simulink model "DCMotorVal"  (R2025a)
settings: Solver=ode23s  StartTime=0.0  StopTime=10  RelTol=1e-3
undefined symbols (not defined in the file): rev_comms_sink
settings Model: Creator=jmp8430  LastModifiedBy=jmp8430

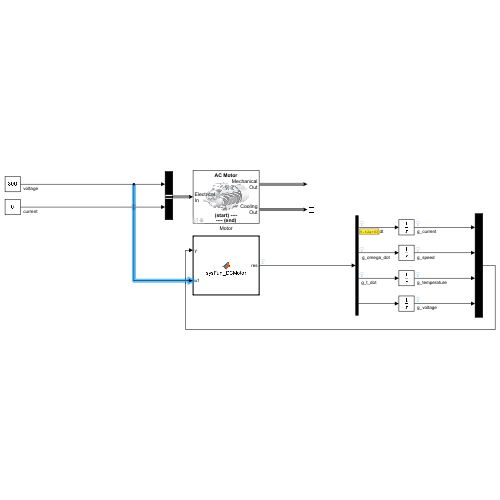
[thumbnail: Simulink's stored preview of the top-level diagram]
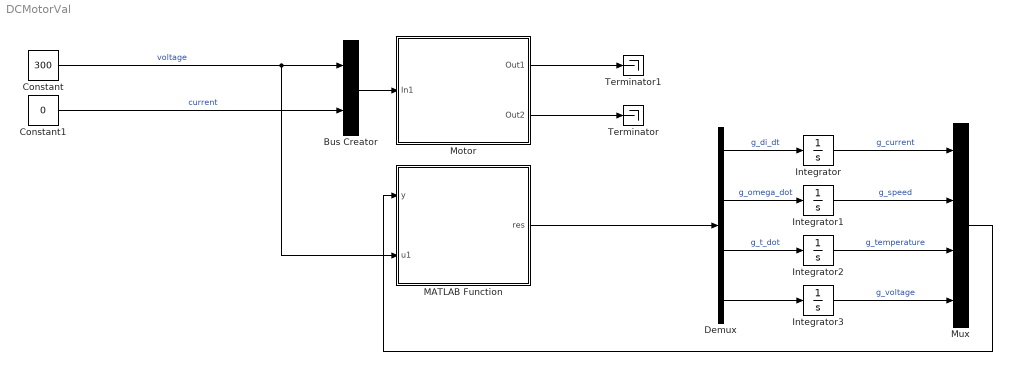
== system DCMotorVal ==
  Bus Creator : BusCreator  Inputs=2
  Constant : Constant  Value=300
  Constant1 : Constant  Value=0
  Demux : Demux
  Integrator : Integrator  InitialCondition=1
  Integrator1 : Integrator  InitialCondition=1
  Integrator2 : Integrator  InitialCondition=25
  Integrator3 : Integrator  InitialCondition=25
  MATLAB Function : MATLAB Function  TreatAsAtomicUnit=on
  Motor : Subsystem  AncestorBlock=DAEMOT_Lib/Electrical/Motor  mask{m_type=AC, R=0.013461960749493, Kv=0.009688163543703, c=0.000234355495215172, b=1.89435163576232e-05, L=1.252192537082724e-05, J=1.09*10^-4, I_initial=1, w_initial=1, Cp=60, T_initial=25}
      mask prompts: m_type "Motor Type"; R "Armature Resistance [Ohm]"; Kv "Motor Constant [Nm/A] or [V-s/rad]"; c "Static Friction Coefficient [Nm]"; b "Viscous Friction Coefficient [N*m*s/rad]"; L "Armature Inductance [H]"; J "Shaft Inertia [kg*m^2]"; I_initial "Initial Total Current [A]"; w_initial "Initial Speed [rad/s]"; Cp "Motor Heat Capacity [J/K]"; T_initial "Initial Temperature [C]"
      settings: LibrarySourceBlock=DAEMOT_Lib_Copy/Dyn Electrical Comp/Motor
      settings: CopyFcn=|
      | h      = get_param(gcb,'handle');   % Get block handle
      | blk    = gcb;
      | 
      | set_param(blk, 'LinkStatus', 'inactive')
      | clear h
      | clear blk
      mask TypeOptions m_type: DC | AC
      mask DialogControl ParameterTabVar0 Prompt: Motor Parameters
      mask DialogControl ParameterTabVar01 Prompt: Cooling
      mask DialogControl ParameterTabVar012 Prompt: System
      mask Display:
      | image(imread('motor.bmp'));
      | T = get_param(gcb,'m_type');
      | if strcmp(T,'DC')
      |     text(0.5,0.95,['{\bf DC Motor}'],'TexMode','on','horizontalAlignment', 'center')
      | else
      |     text(0.5,0.95,['{\bf AC Motor}'],'TexMode','on','horizontalAlignment', 'center')
      | end
      | text(0.5,0.075,['{\bf ---- (end)}'],'TexMode','on','horizontalAlignment', 'center')
      | text(0.5,0.175,['{\bf (start) ----}'],'TexMode','on','horizontalAlignment', 'center')
      | 
      | port_label('input',1,sprintf('Electrical \nIn'))
      | port_label('output',1,sprintf('Mechanical \nOut'))
      | port_label('output',2,sprintf('Cooling \nOut'))
  Mux : Mux
  Terminator : Terminator
  Terminator1 : Terminator
  wires:
  MATLAB Function/1(res) -> Demux/1
  Motor/2(Out2) -> Terminator/1
  Motor/1(Out1) -> Terminator1/1
  Constant/1 -> MATLAB Function/2(u1), Bus Creator/1  "voltage"
  Bus Creator/1 -> Motor/1(In1)
  Constant1/1 -> Bus Creator/2  "current"
  Demux/1 -> Integrator/1  "g_di_dt"
  Demux/2 -> Integrator1/1  "g_omega_dot"
  Demux/3 -> Integrator2/1  "g_t_dot"
  Demux/4 -> Integrator3/1
  Integrator/1 -> Mux/1  "g_current"
  Integrator1/1 -> Mux/2  "g_speed"
  Integrator2/1 -> Mux/3  "g_temperature"
  Mux/1 -> MATLAB Function/1(y)
  Integrator3/1 -> Mux/4  "g_voltage"

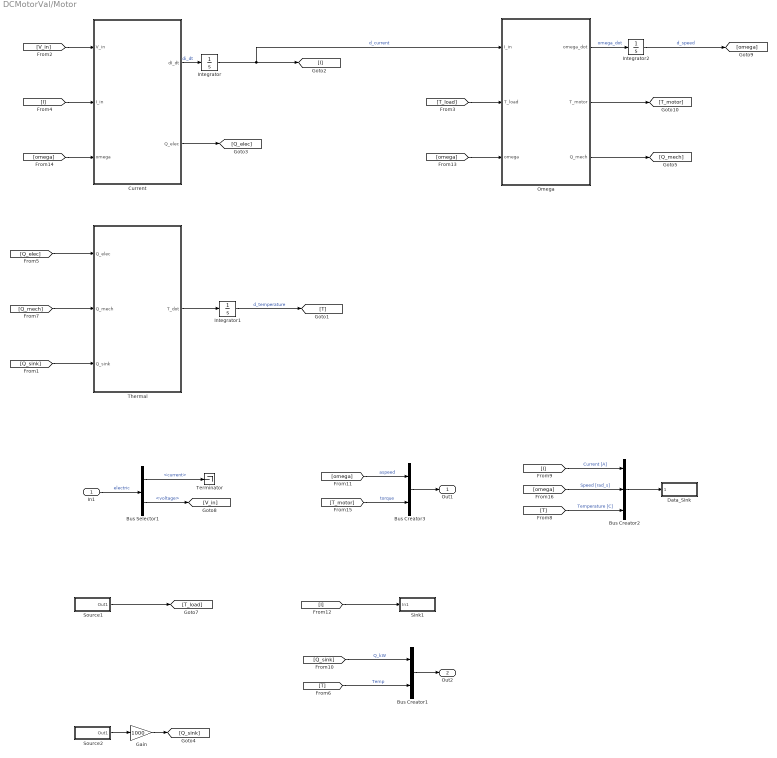
== system DCMotorVal/Motor ==
  In1 : Inport
  Bus Creator1 : BusCreator  Inputs=2
  Bus Creator2 : BusCreator  Inputs=3
  Bus Creator3 : BusCreator  Inputs=2
  Bus Selector1 : BusSelector  OutputSignals=current,voltage
  Current : MATLAB Function  TreatAsAtomicUnit=on
  Data_Sink : Subsystem  LoadFcn=|  InitFcn=|  mask(Data Sink){}
      LoadFcn=|
      | h      = get_param(gcb,'handle');   % Get block handle                           
      | hblock = get(h);     % Parse out handles structure
      | 
      | str = [hblock.Path(numel(bdroot)+2:end), hblock.Name];
      | str(~ismember(str,['A':'Z' 'a':'z' '0':'9' '_'])) = '';                     
      | set_param([gcb, '/global_data_goto'],'GotoTag',['gdata_',str]);
      |                                
      |                                                                                  
      | clear h hblock str
      InitFcn=|
      | h      = get_param(gcb,'handle');   % Get block handle                           
      | hblock = get(h);     % Parse out handles structure
      | 
      | str = [hblock.Path(numel(bdroot)+2:end), hblock.Name];
      | str(~ismember(str,['A':'Z' 'a':'z' '0':'9' '_'])) = '';                     
      | set_param([gcb, '/global_data_goto'],'GotoTag',['gdata_',str]);
      |                                
      |                                                                                  
      | clear h hblock str
      mask help:
      | Input to this block should be a bus signal with named signals.
      |
      | Bus signals sent to this block will be read by the Data Manager.
      | The Data Manager will handle the global routing of signals.
      |
      | This block should be placed under the mask of components.
      settings: CopyFcn=|
      | h      = get_param(gcb,'handle');   % Get block handle
      | hblock = get(h);     % Parse out handles structure
      | 
      | str = [hblock.Path(numel(bdroot)+2:end), hblock.Name];
      | str(~ismember(str,['A':'Z' 'a':'z' '0':'9' '_'])) = '';
      | set_param([gcb, '/global_data_goto'],'GotoTag',['gdata_',str]);
      | 
      | 
      | clear h hblock str
      settings: NameChangeFcn=|
      | h      = get_param(gcb,'handle');   % Get block handle
      | hblock = get(h);     % Parse out handles structure
      | 
      | str = [hblock.Path(numel(bdroot)+2:end), hblock.Name];
      | str(~ismember(str,['A':'Z' 'a':'z' '0':'9' '_'])) = '';
      | set_param([gcb, '/global_data_goto'],'GotoTag',['gdata_',str]);
      | 
      | 
      | clear h hblock str
      mask Display: text(0.25,0.5,'Data Sink')
  Gain : Gain  Gain=1000
  Integrator : Integrator  InitialCondition=I_initial
  Integrator1 : Integrator  InitialCondition=T_initial
  Integrator2 : Integrator  InitialCondition=w_initial
  Omega : MATLAB Function  TreatAsAtomicUnit=on
  Sink1 : Subsystem  LoadFcn=rev_comms_sink();  InitFcn=rev_comms_sink();  mask(Sink){}
      mask help: Used for sending data to the upstream component.
      settings: CopyFcn=rev_comms_sink();  NameChangeFcn=rev_comms_sink();
      mask Display: text(0.25,0.5,'Sink')
  Source1 : Subsystem  mask(Source){}
      mask help: Used for receiving data from the downstream component.
      mask init:
      | n_src = gcb;
      | n_src = str2num(n_src(end));
      | try
      |     rev_comms_source(n_src);
      | catch
      | 
      | end
      mask Display: text(0.25,0.5,'Source')
  Source2 : Subsystem  mask(Source){}
      mask help: Used for receiving data from the downstream component.
      mask init:
      | n_src = gcb;
      | n_src = str2num(n_src(end));
      | try
      |     rev_comms_source(n_src);
      | catch
      | 
      | end
      mask Display: text(0.25,0.5,'Source')
  Terminator : Terminator
  Thermal : MATLAB Function  TreatAsAtomicUnit=on
  Out1 : Outport
  Out2 : Outport  Port=2
  wires:
  Gain/1 -> [Q_sink]
  [Q_sink] -> Bus Creator1/1  "Q_kW"
  [T] -> Bus Creator1/2  "Temp"
  Bus Creator1/1 -> Out2/1
  [Q_mech] -> Thermal/2(Q_mech)
  Omega/3(Q_mech) -> [Q_mech]
  [omega] -> Omega/3(omega)
  Source1/1(Out1) -> [T_load]
  Source2/1(Out1) -> Gain/1
  [V_in] -> Current/1(V_in)
  Integrator/1 -> [I], Omega/1(I_in)  "d_current"
  [T] -> Bus Creator2/3  "Temperature [C]"
  [omega] -> Bus Creator2/2  "Speed [rad_s]"
  Bus Creator2/1 -> Data_Sink/1(" ")
  [omega] -> Current/3(omega)
  Bus Selector1/1 -> Terminator/1  "<current>"
  Bus Selector1/2 -> [V_in]  "<voltage>"
  [omega] -> Bus Creator3/1  "aspeed"
  [I] -> Sink1/1(In1)
  In1/1 -> Bus Selector1/1  "electric"
  Bus Creator3/1 -> Out1/1
  Current/1(dI_dt) -> Integrator/1  "di_dt"
  [I] -> Current/2(I_in)
  Thermal/1(T_dot) -> Integrator1/1
  Integrator1/1 -> [T]  "d_temperature"
  Current/2(Q_elec) -> [Q_elec]
  [Q_elec] -> Thermal/1(Q_elec)
  [Q_sink] -> Thermal/3(Q_sink)
  Omega/1(omega_dot) -> Integrator2/1  "omega_dot"
  [T_load] -> Omega/2(T_load)
  Integrator2/1 -> [omega]  "d_speed"
  Omega/2(T_motor) -> [T_motor]
  [T_motor] -> Bus Creator3/2  "torque"
  [I] -> Bus Creator2/1  "Current [A]"

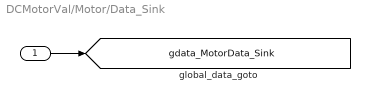
== system DCMotorVal/Motor/Data_Sink ==
  " " : Inport
  tag scope: gdata_MotorData_Sink=global
  wires:
  " "/1 -> [gdata_MotorData_Sink]

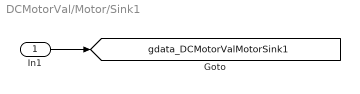
== system DCMotorVal/Motor/Sink1 ==
  In1 : Inport
  tag scope: gdata_DCMotorValMotorSink1=global
  wires:
  In1/1 -> [gdata_DCMotorValMotorSink1]

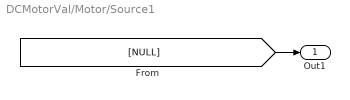
== system DCMotorVal/Motor/Source1 ==
  Out1 : Outport
  wires:
  [NULL] -> Out1/1

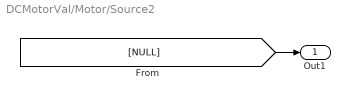
== system DCMotorVal/Motor/Source2 ==
  Out1 : Outport
  wires:
  [NULL] -> Out1/1

== matlab function DCMotorVal/MATLAB Function ==
  data: res output; y input; u1 input
function res = sysFun_DCMotor(y,u1)
J = 0.000109;
Cp = 60;
L = 1.25219e-05;
b = 1.89435e-05;
c = 0.000234355;
R = 0.013462;
Kt = 0.00968816;
x1 = y(1);
x2 = y(2);
x3 = y(3);
x4 = y(4);
x1_dot = (1/(L*x1))*(-(Kt*x1*x2)-(R*x1^2)+(x1*u1));
x2_dot = (1/(J*x2))*(+(Kt*x1*x2)-(b*x2^2+c*x2));
x3_dot = (1/(Cp))*(+(b*x2^2+c*x2)+(R*x1^2));
x4_dot = 0;
res = [x1_dot;x2_dot;x3_dot;x4_dot];
end

== matlab function DCMotorVal/Motor/Current ==
  data: V_in input; I_in input; Kv parameter; R parameter; L parameter; omega input; dI_dt output; Q_elec output
function [dI_dt,Q_elec]= current(V_in,I_in,Kv, R, L,omega)


dI_dt = (1/L) * (V_in - R*I_in - Kv*omega);

Q_elec = R*I_in^2;

== matlab function DCMotorVal/Motor/Omega ==
  data: I_in input; T_load input; omega_dot output; Kv parameter; omega input; T_motor output; J parameter; b parameter; c parameter; Q_mech output
function [omega_dot,T_motor,Q_mech]= omega(I_in,T_load,Kv,omega,J, b,c)

T_motor = Kv*I_in;

omega_dot = (1/(J))*(T_motor - T_load - b*omega - c*(2./(1+exp(-5*omega)) - 1));
Q_mech = b*omega^2 + c*omega*(2./(1+exp(-5*omega)) - 1);

== matlab function DCMotorVal/Motor/Thermal ==
  data: Q_elec input; Q_mech input; T_dot output; Q_sink input; Cp parameter
function T_dot = Thermal(Q_elec,Q_mech, Q_sink, Cp)
%% Load Temperature
T_dot = (1/Cp) * (Q_elec + Q_mech - Q_sink);
